simulink model "pulse24rectifier"  (R2023b)
settings: Solver=VariableStepAuto  StartTime=0.0  StopTime=0.3  RelTol=1e-3
undefined symbols (not defined in the file): D1, lagging, pulse
libraries: spsPLL3phLib x4, spsPulseGeneratorThyristor6PulseLib x4, spsUniversalBridgeLib x4, spsZigzagPhaseShiftingTransformerLib x4, spsSeriesRLCBranchLib x3, spsVoltageMeasurementLib x2, spsRMSLib x1, spsThreePhaseVIMeasurementLib x1, spsThreePhaseSourceLib x1, sps_lib x1
settings Model: Creator=memos  LastModifiedBy=memos

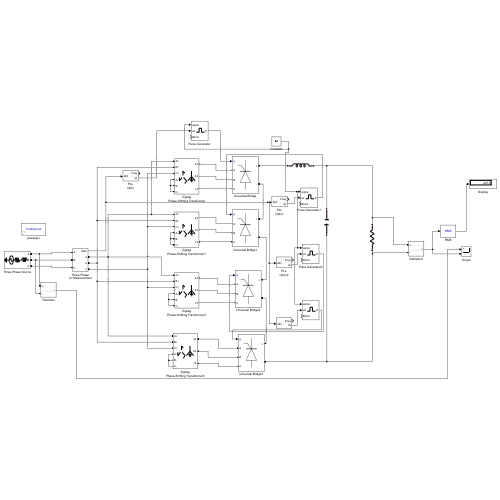
[thumbnail: Simulink's stored preview of the top-level diagram]
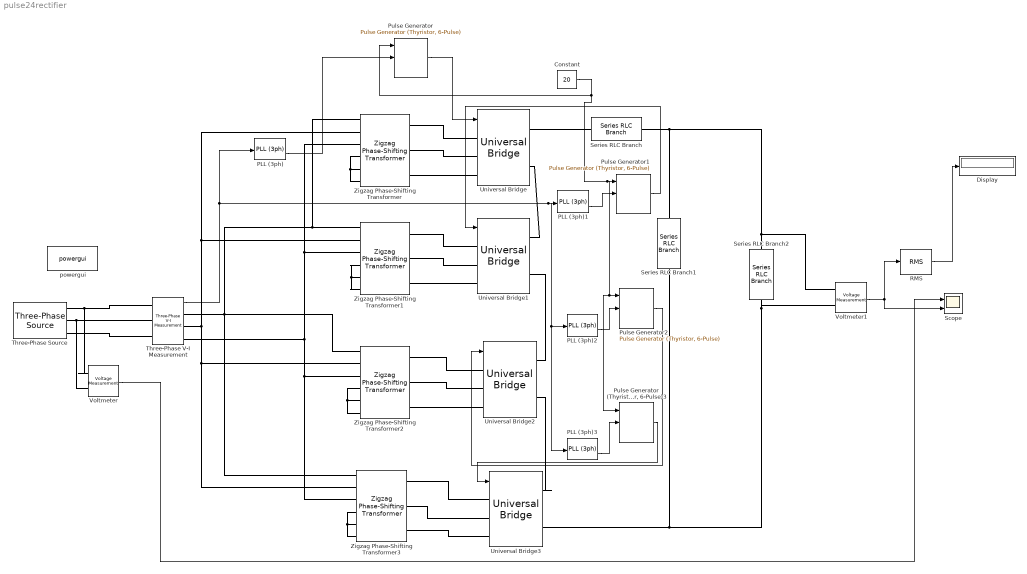
== system pulse24rectifier ==
  Constant : Constant  Value=20
  Display : Display
  PLL (3ph){,1..3} (4 alike) : spsPLL3phLib/PLL (3ph)  Fmin=45  Par_Init=[0, 60]  ParK=[180, 3200, 1]  TcD=1e-4  MaxRateChangeFreq=12  FilterCutOffFreq=25  Ts=0  AGC=on
  Pulse Generator : spsPulseGeneratorThyristor6PulseLib/Pulse Generator (Thyristor, 6-Pulse)  GenType=6-pulse  Delta=D1 (lagging)  pwidth=90  Double_Pulse=off  Ts=0
      settings: LibrarySourceBlock=|
      | sps_lib/Power Electronics/Power Electronics Control/Pulse Generator
      | (Thyristor, 6-Pulse)
  "Pulse Generator (Thyristor, 6-Pulse)3" : spsPulseGeneratorThyristor6PulseLib/Pulse Generator (Thyristor, 6-Pulse)  GenType=6-pulse  Delta=D1 (lagging)  pwidth=90  Double_Pulse=off  Ts=0
      settings: LibrarySourceBlock=|
      | sps_lib/Power Electronics/Power Electronics Control/Pulse Generator
      | (Thyristor, 6-Pulse)
  Pulse Generator1 : spsPulseGeneratorThyristor6PulseLib/Pulse Generator (Thyristor, 6-Pulse)  GenType=6-pulse  Delta=D1 (lagging)  pwidth=90  Double_Pulse=off  Ts=0
      settings: LibrarySourceBlock=|
      | sps_lib/Power Electronics/Power Electronics Control/Pulse Generator
      | (Thyristor, 6-Pulse)
  Pulse Generator2 : spsPulseGeneratorThyristor6PulseLib/Pulse Generator (Thyristor, 6-Pulse)  GenType=6-pulse  Delta=D1 (lagging)  pwidth=90  Double_Pulse=off  Ts=0
      settings: LibrarySourceBlock=|
      | sps_lib/Power Electronics/Power Electronics Control/Pulse Generator
      | (Thyristor, 6-Pulse)
  RMS : spsRMSLib/RMS  TrueRMS=on  Freq=50  RMSInit=120  Ts=0
  Scope : Scope  NumInputPorts=2
  Series RLC Branch : spsSeriesRLCBranchLib/Series RLC Branch  LConnTagsString=__new0  RConnTagsString=__new0  BranchType=L  Resistance=1  Inductance=200e-3  SetiL0=off  InitialCurrent=0  Capacitance=1e-6  Setx0=off  InitialVoltage=0  Measurements=None
  Series RLC Branch1 : spsSeriesRLCBranchLib/Series RLC Branch  LConnTagsString=__new0  RConnTagsString=__new0  BranchType=C  Resistance=1  Inductance=200e-3  SetiL0=off  InitialCurrent=0  Capacitance=10e-6  Setx0=off  InitialVoltage=0  Measurements=None
  Series RLC Branch2 : spsSeriesRLCBranchLib/Series RLC Branch  LConnTagsString=__new0  RConnTagsString=__new0  BranchType=R  Resistance=1400  Inductance=200e-3  SetiL0=off  InitialCurrent=0  Capacitance=1e-6  Setx0=off  InitialVoltage=0  Measurements=None
  Three-Phase V-I Measurement : spsThreePhaseVIMeasurementLib/Three-Phase V-I Measurement  VoltageMeasurement=phase-to-ground  SetLabelV=off  LabelV=Vabc  Vpu=off  VpuLL=off  CurrentMeasurement=no  SetLabelI=off  LabelI=Iabc  Ipu=off  Pbase=100e6  Vbase=500e3  OutputType=Complex  PhasorSimulation=off  PSBequivalent=0
  Three-Phase Source : spsThreePhaseSourceLib/Three-Phase Source  InternalConnection=Yg  VoltagePhases=off  Voltage=254.05  PhaseAngle=0  Voltage_phases=[25e3 25e3 25e3]/sqrt(3)  PhaseAngles_phases=[0 -120 +120]  Frequency=50  NonIdealSource=on  SpecifyImpedance=off  Resistance=0.8929  Inductance=16.58e-3  ShortCircuitLevel=100e6  BaseVoltage=25e3  XRratio=7  BusType=swing  Pref=10e3  Qref=0  Prefabc=[10e3, 10e3, 10e3]  Qrefabc=[0, 0, 0]  Qmin=-inf  Qmax=inf
  Universal Bridge{,1..3} (4 alike) : spsUniversalBridgeLib/Universal Bridge  Arms=3  SnubberResistance=1e5  SnubberCapacitance=inf  Device=Thyristors  Ron=1e-3  Lon=0  ForwardVoltages="[  0  0  ]"  ForwardVoltage=0  GTOparameters=[ 10e-6 , 20e-6 ]  IGBTparameters=[ 1e-6 , 2e-6 ]  Measurements=None  Measurements_2=None  converterType=Rectifier
  Voltmeter : spsVoltageMeasurementLib/Voltage Measurement  PhasorSimulation=off  OutputType=Complex  PSBequivalent=0
  Voltmeter1 : spsVoltageMeasurementLib/Voltage Measurement  PhasorSimulation=off  OutputType=Complex  PSBequivalent=0
  Zigzag Phase-Shifting Transformer{,1..3} (4 alike) : spsZigzagPhaseShiftingTransformerLib/Zigzag Phase-Shifting Transformer  SecondaryConnection=Yg  SetSaturation=off  SetInitialFlux=off  Measurements=None  UNITS=pu  NominalPower=[ 50e3 50]  PrimaryVoltage=10e3  SecondaryVoltage="[ 30e3  +15]"  Winding1=[ 0.002 0.08 ]  Winding2="[ 0.002  0.08 ]"  Winding3=[ 0.002 0.08 ]  RmLm=[ 500 500 ]  Rm=500  Saturation=[ 0,0 ; 0.0024,1.2 ; 1.0,1.52 ]  InitialFluxes=[0,0,0]  BreakLoop=off  DiscreteSolver=Trapezoidal iterative  DataType=off
      settings: LibrarySourceBlock=|
      | sps_lib/Power Grid Elements/Zigzag
      | Phase-Shifting Transformer
  powergui : sps_lib/powergui  Priority=1  SimulationMode=Continuous  SampleTime=50e-6  frequency=60  Iterations=50  frequencyindice=50  Pbase=100e6  ErrMax=1e-4  UnitsV=kV  UnitsW=MW  buscounter=0  FunctionMessages=off  echomessages=off  EnableUseOfTLC=off  CurrentSourceSwitches=off  DisableSnubberDevices=off  DisableRonSwitches=off  DisableVfSwitches=off  DisplayEquations=off  AutomaticDiscreteSolvers=off  SolverType=Tustin/Backward Euler (TBE)  Interpol=off  ExternalGateDelay=off  methode=off  Ts=100  x0status=blocks  SPID=on  SwTol=0  HookPort=off  NonlinearTolerance=1e-4  nMaxIteration=100  ContinueOnMaxIteration=off  RestoreLinks=warning  ResistiveCurrentMeasurement=off  Frange=[0:2:500]  Ylog=off  Xlog=on  ShowGrid=off  save=off  variable=ZData  structure=0  ZoomFFT=off  StartTime=0.0  cycles=1  DisplayStyle=1  fundamental=60  FreqAxis=off  MaxFrequency=1000  frequencyindicesteady=1  RmsSteady=1  display=off
  wires:
  Three-Phase V-I Measurement/1 -> PLL (3ph)/1, PLL (3ph)3/1, PLL (3ph)2/1, PLL (3ph)1/1
  PLL (3ph)/2 -> Pulse Generator/2
  Voltmeter1/1 -> Scope/2, RMS/1
  RMS/1 -> Display/1
  Constant/1 -> "Pulse Generator (Thyristor, 6-Pulse)3"/1, Pulse Generator2/1, Pulse Generator1/1, Pulse Generator/1
  PLL (3ph)1/2 -> Pulse Generator1/2
  PLL (3ph)2/2 -> Pulse Generator2/2
  PLL (3ph)3/2 -> "Pulse Generator (Thyristor, 6-Pulse)3"/2
  Pulse Generator/1 -> Universal Bridge/1
  Pulse Generator1/1 -> Universal Bridge1/1
  Pulse Generator2/1 -> Universal Bridge2/1
  "Pulse Generator (Thyristor, 6-Pulse)3"/1 -> Universal Bridge3/1
  Voltmeter/1 -> Scope/1
  connections:
  Three-Phase Source/RConn1 -- Voltmeter/LConn1 -- Three-Phase V-I Measurement/LConn1
  Three-Phase Source/RConn2 -- Voltmeter/LConn2 -- Three-Phase V-I Measurement/LConn2
  Three-Phase Source/RConn3 -- Three-Phase V-I Measurement/LConn3
  Zigzag Phase-Shifting Transformer/LConn4 -- Zigzag Phase-Shifting Transformer/LConn5 -- Zigzag Phase-Shifting Transformer/LConn6
  Zigzag Phase-Shifting Transformer1/LConn4 -- Zigzag Phase-Shifting Transformer1/LConn6 -- Zigzag Phase-Shifting Transformer1/LConn5
  Zigzag Phase-Shifting Transformer2/LConn4 -- Zigzag Phase-Shifting Transformer2/LConn5 -- Zigzag Phase-Shifting Transformer2/LConn6
  Zigzag Phase-Shifting Transformer3/LConn4 -- Zigzag Phase-Shifting Transformer3/LConn6 -- Zigzag Phase-Shifting Transformer3/LConn5
  Three-Phase V-I Measurement/RConn3 -- Zigzag Phase-Shifting Transformer3/LConn3 -- Zigzag Phase-Shifting Transformer2/LConn3 -- Zigzag Phase-Shifting Transformer1/LConn3 -- Zigzag Phase-Shifting Transformer/LConn3
  Three-Phase V-I Measurement/RConn2 -- Zigzag Phase-Shifting Transformer3/LConn2 -- Zigzag Phase-Shifting Transformer2/LConn2 -- Zigzag Phase-Shifting Transformer/LConn2 -- Zigzag Phase-Shifting Transformer1/LConn2
  Zigzag Phase-Shifting Transformer2/LConn1 -- Zigzag Phase-Shifting Transformer/LConn1 -- Zigzag Phase-Shifting Transformer1/LConn1 -- Three-Phase V-I Measurement/RConn1 -- Zigzag Phase-Shifting Transformer3/LConn1
  Zigzag Phase-Shifting Transformer/RConn1 -- Universal Bridge/LConn1
  Zigzag Phase-Shifting Transformer/RConn2 -- Universal Bridge/LConn2
  Zigzag Phase-Shifting Transformer/RConn3 -- Universal Bridge/LConn3
  Zigzag Phase-Shifting Transformer1/RConn1 -- Universal Bridge1/LConn1
  Universal Bridge1/LConn2 -- Zigzag Phase-Shifting Transformer1/RConn2
  Zigzag Phase-Shifting Transformer1/RConn3 -- Universal Bridge1/LConn3
  Zigzag Phase-Shifting Transformer2/RConn1 -- Universal Bridge2/LConn1
  Zigzag Phase-Shifting Transformer2/RConn2 -- Universal Bridge2/LConn2
  Zigzag Phase-Shifting Transformer2/RConn3 -- Universal Bridge2/LConn3
  Zigzag Phase-Shifting Transformer3/RConn1 -- Universal Bridge3/LConn1
  Zigzag Phase-Shifting Transformer3/RConn2 -- Universal Bridge3/LConn2
  Zigzag Phase-Shifting Transformer3/RConn3 -- Universal Bridge3/LConn3
  Universal Bridge1/RConn1 -- Universal Bridge/RConn2
  Universal Bridge1/RConn2 -- Universal Bridge2/RConn1
  Universal Bridge3/RConn1 -- Universal Bridge2/RConn2
  Series RLC Branch/LConn1 -- Universal Bridge/RConn1
  Series RLC Branch/RConn1 -- Voltmeter1/LConn1 -- Series RLC Branch2/LConn1 -- Series RLC Branch1/LConn1
  Universal Bridge3/RConn2 -- Voltmeter1/LConn2 -- Series RLC Branch2/RConn1 -- Series RLC Branch1/RConn1
